simulink model "RADTRANS002"  (R2020b)
settings: Solver=VariableStepAuto  StartTime=0.0  StopTime=10.0  RelTol=1e-3
undefined symbols (not defined in the file): Line_110_C, Line_110_L, Line_110_R, Line_220_C, Line_220_L, Line_220_R, Line_35_C, Line_35_L, Line_35_R, Line_6_L, Line_6_R, Sys_f_Hz, Sys_V_net_kV, Tr_110_35_L_pu, Tr_110_35_R_pu, Tr_110_35_Sn_VA, Tr_110_35_V_HV_kV, Tr_110_35_V_LV_kV, Tr_110_6_L_pu, Tr_110_6_R_pu, Tr_110_6_Sn_VA, Tr_110_6_V_HV_kV, Tr_110_6_V_LV_kV, Tr_220_110_L_pu, Tr_220_110_R_pu, Tr_220_110_Sn_VA, Tr_220_110_V_HV_kV, Tr_220_110_V_LV_kV, Tr_35_04_L_pu, Tr_35_04_R_pu, Tr_35_04_Sn_VA, Tr_35_04_V_HV_kV, Tr_35_04_V_LV_kV, Tr_6_04_L_pu, Tr_6_04_R_pu, Tr_6_04_Sn_VA, Tr_6_04_V_HV_kV, Tr_6_04_V_LV_kV, Ts_powergui
libraries: dspstat3 x288, powerlib x202, powerlib_meascontrol x72
(part 7 of 7)

== system RADTRANS002/M_OUT_Завод_5_1 ==
  Iptg_50 : Display
      settings: Format=bank
  PQptg_50 : Scope  NumInputPorts=2
  "Power0 (3ph, Instantaneous)" : powerlib_meascontrol/Measurements/Power (3ph, Instantaneous)
  Pptg_50 : Display
      settings: Format=bank
  Qptg_50 : Display
      settings: Format=bank
  RMS3 : dspstat3/RMS  run=off  directionMode=Each column  dimension=1  InputProcessing=Columns as channels (frame based)  reset_popup=None
  RMS4 : dspstat3/RMS  run=off  directionMode=Each column  dimension=1  InputProcessing=Columns as channels (frame based)  reset_popup=None
  RMS50 : dspstat3/RMS  run=off  directionMode=Each column  dimension=1  InputProcessing=Columns as channels (frame based)  reset_popup=None
  RMSpt_50 : dspstat3/RMS  run=off  directionMode=Each column  dimension=1  InputProcessing=Columns as channels (frame based)  reset_popup=None
  Real-Ima to Complex : RealImagToComplex
  S : Abs
  SSptg_50 : Scope
  Sptg_50 : Display
      settings: Format=bank
  Three-Phase V-I Measurementpt_50 : powerlib/Measurements/Three-Phase V-I Measurement  VoltageMeasurement=phase-to-ground  SetLabelV=off  LabelV=Vabc  Vpu=off  VpuLL=off  CurrentMeasurement=yes  SetLabelI=off  LabelI=Iabc  Ipu=off  Pbase=100e6  Vbase=500e3  OutputType=Complex  PhasorSimulation=off  PSBequivalent=0
  UIptg_50 : Scope  NumInputPorts=2
  Uptg_50 : Display
      settings: Format=bank
  a : PMIOPort  Side=Right
  b : PMIOPort  Port=2  Side=Right
  c : PMIOPort  Port=3  Side=Right
  A : PMIOPort  Port=4  Side=Left
  B : PMIOPort  Port=5  Side=Left
  C : PMIOPort  Port=6  Side=Left
  tag scope: I_ptg_50=global, P_ptg_50=global, Q_ptg_50=global, S_ptg_50=global, U_ptg_50=global
  wires:
  S/1 -> [S_ptg_50]
  Real-Ima to Complex/1 -> S/1
  [S_ptg_50] -> Sptg_50/1
  [S_ptg_50] -> SSptg_50/1
  [P_ptg_50] -> RMSpt_50/1
  RMSpt_50/1 -> Pptg_50/1
  RMS50/1 -> Qptg_50/1
  [U_ptg_50] -> RMS3/1
  RMS3/1 -> Uptg_50/1
  [P_ptg_50] -> Real-Ima to Complex/1
  [Q_ptg_50] -> RMS50/1
  [I_ptg_50] -> RMS4/1
  RMS4/1 -> Iptg_50/1
  [U_ptg_50] -> UIptg_50/1  "U"
  [P_ptg_50] -> PQptg_50/1  "P"
  [I_ptg_50] -> UIptg_50/2  "I"
  Three-Phase V-I Measurementpt_50/1 -> [U_ptg_50]
  [Q_ptg_50] -> Real-Ima to Complex/2
  Three-Phase V-I Measurementpt_50/2 -> [I_ptg_50]
  [U_ptg_50] -> "Power0 (3ph, Instantaneous)"/1
  [I_ptg_50] -> "Power0 (3ph, Instantaneous)"/2
  "Power0 (3ph, Instantaneous)"/2 -> [Q_ptg_50]
  "Power0 (3ph, Instantaneous)"/1 -> [P_ptg_50]
  [Q_ptg_50] -> PQptg_50/2  "Q"
  connections:
  Three-Phase V-I Measurementpt_50/LConn1 -- A/RConn1
  Three-Phase V-I Measurementpt_50/RConn1 -- a/RConn1
  Three-Phase V-I Measurementpt_50/LConn2 -- B/RConn1
  Three-Phase V-I Measurementpt_50/LConn3 -- C/RConn1
  Three-Phase V-I Measurementpt_50/RConn3 -- c/RConn1
  Three-Phase V-I Measurementpt_50/RConn2 -- b/RConn1

== system RADTRANS002/M_OUT_Завод_5_2 ==
  Iptg_52 : Display
      settings: Format=bank
  PQptg_52 : Scope  NumInputPorts=2
  "Power0 (3ph, Instantaneous)" : powerlib_meascontrol/Measurements/Power (3ph, Instantaneous)
  Pptg_52 : Display
      settings: Format=bank
  Qptg_52 : Display
      settings: Format=bank
  RMS3 : dspstat3/RMS  run=off  directionMode=Each column  dimension=1  InputProcessing=Columns as channels (frame based)  reset_popup=None
  RMS4 : dspstat3/RMS  run=off  directionMode=Each column  dimension=1  InputProcessing=Columns as channels (frame based)  reset_popup=None
  RMS52 : dspstat3/RMS  run=off  directionMode=Each column  dimension=1  InputProcessing=Columns as channels (frame based)  reset_popup=None
  RMSpt_52 : dspstat3/RMS  run=off  directionMode=Each column  dimension=1  InputProcessing=Columns as channels (frame based)  reset_popup=None
  Real-Ima to Complex : RealImagToComplex
  S : Abs
  SSptg_52 : Scope
  Sptg_52 : Display
      settings: Format=bank
  Three-Phase V-I Measurementpt_52 : powerlib/Measurements/Three-Phase V-I Measurement  VoltageMeasurement=phase-to-ground  SetLabelV=off  LabelV=Vabc  Vpu=off  VpuLL=off  CurrentMeasurement=yes  SetLabelI=off  LabelI=Iabc  Ipu=off  Pbase=100e6  Vbase=500e3  OutputType=Complex  PhasorSimulation=off  PSBequivalent=0
  UIptg_52 : Scope  NumInputPorts=2
  Uptg_52 : Display
      settings: Format=bank
  a : PMIOPort  Side=Right
  b : PMIOPort  Port=2  Side=Right
  c : PMIOPort  Port=3  Side=Right
  A : PMIOPort  Port=4  Side=Left
  B : PMIOPort  Port=5  Side=Left
  C : PMIOPort  Port=6  Side=Left
  tag scope: I_ptg_52=global, P_ptg_52=global, Q_ptg_52=global, S_ptg_52=global, U_ptg_52=global
  wires:
  S/1 -> [S_ptg_52]
  Real-Ima to Complex/1 -> S/1
  [S_ptg_52] -> Sptg_52/1
  [S_ptg_52] -> SSptg_52/1
  [P_ptg_52] -> RMSpt_52/1
  RMSpt_52/1 -> Pptg_52/1
  RMS52/1 -> Qptg_52/1
  [U_ptg_52] -> RMS3/1
  RMS3/1 -> Uptg_52/1
  [P_ptg_52] -> Real-Ima to Complex/1
  [Q_ptg_52] -> RMS52/1
  [I_ptg_52] -> RMS4/1
  RMS4/1 -> Iptg_52/1
  [U_ptg_52] -> UIptg_52/1  "U"
  [P_ptg_52] -> PQptg_52/1  "P"
  [I_ptg_52] -> UIptg_52/2  "I"
  Three-Phase V-I Measurementpt_52/1 -> [U_ptg_52]
  [Q_ptg_52] -> Real-Ima to Complex/2
  Three-Phase V-I Measurementpt_52/2 -> [I_ptg_52]
  [U_ptg_52] -> "Power0 (3ph, Instantaneous)"/1
  [I_ptg_52] -> "Power0 (3ph, Instantaneous)"/2
  "Power0 (3ph, Instantaneous)"/2 -> [Q_ptg_52]
  "Power0 (3ph, Instantaneous)"/1 -> [P_ptg_52]
  [Q_ptg_52] -> PQptg_52/2  "Q"
  connections:
  Three-Phase V-I Measurementpt_52/LConn1 -- A/RConn1
  Three-Phase V-I Measurementpt_52/RConn1 -- a/RConn1
  Three-Phase V-I Measurementpt_52/LConn2 -- B/RConn1
  Three-Phase V-I Measurementpt_52/LConn3 -- C/RConn1
  Three-Phase V-I Measurementpt_52/RConn3 -- c/RConn1
  Three-Phase V-I Measurementpt_52/RConn2 -- b/RConn1

== system RADTRANS002/M_OUT_Завод_6_1 ==
  Iptg_62 : Display
      settings: Format=bank
  PQptg_62 : Scope  NumInputPorts=2
  "Power0 (3ph, Instantaneous)" : powerlib_meascontrol/Measurements/Power (3ph, Instantaneous)
  Pptg_62 : Display
      settings: Format=bank
  Qptg_62 : Display
      settings: Format=bank
  RMS3 : dspstat3/RMS  run=off  directionMode=Each column  dimension=1  InputProcessing=Columns as channels (frame based)  reset_popup=None
  RMS4 : dspstat3/RMS  run=off  directionMode=Each column  dimension=1  InputProcessing=Columns as channels (frame based)  reset_popup=None
  RMS62 : dspstat3/RMS  run=off  directionMode=Each column  dimension=1  InputProcessing=Columns as channels (frame based)  reset_popup=None
  RMSpt_62 : dspstat3/RMS  run=off  directionMode=Each column  dimension=1  InputProcessing=Columns as channels (frame based)  reset_popup=None
  Real-Ima to Complex : RealImagToComplex
  S : Abs
  SSptg_62 : Scope
  Sptg_62 : Display
      settings: Format=bank
  Three-Phase V-I Measurementpt_62 : powerlib/Measurements/Three-Phase V-I Measurement  VoltageMeasurement=phase-to-ground  SetLabelV=off  LabelV=Vabc  Vpu=off  VpuLL=off  CurrentMeasurement=yes  SetLabelI=off  LabelI=Iabc  Ipu=off  Pbase=100e6  Vbase=500e3  OutputType=Complex  PhasorSimulation=off  PSBequivalent=0
  UIptg_62 : Scope  NumInputPorts=2
  Uptg_62 : Display
      settings: Format=bank
  a : PMIOPort  Side=Right
  b : PMIOPort  Port=2  Side=Right
  c : PMIOPort  Port=3  Side=Right
  A : PMIOPort  Port=4  Side=Left
  B : PMIOPort  Port=5  Side=Left
  C : PMIOPort  Port=6  Side=Left
  tag scope: I_ptg_62=global, P_ptg_62=global, Q_ptg_62=global, S_ptg_62=global, U_ptg_62=global
  wires:
  S/1 -> [S_ptg_62]
  Real-Ima to Complex/1 -> S/1
  [S_ptg_62] -> Sptg_62/1
  [S_ptg_62] -> SSptg_62/1
  [P_ptg_62] -> RMSpt_62/1
  RMSpt_62/1 -> Pptg_62/1
  RMS62/1 -> Qptg_62/1
  [U_ptg_62] -> RMS3/1
  RMS3/1 -> Uptg_62/1
  [P_ptg_62] -> Real-Ima to Complex/1
  [Q_ptg_62] -> RMS62/1
  [I_ptg_62] -> RMS4/1
  RMS4/1 -> Iptg_62/1
  [U_ptg_62] -> UIptg_62/1  "U"
  [P_ptg_62] -> PQptg_62/1  "P"
  [I_ptg_62] -> UIptg_62/2  "I"
  Three-Phase V-I Measurementpt_62/1 -> [U_ptg_62]
  [Q_ptg_62] -> Real-Ima to Complex/2
  Three-Phase V-I Measurementpt_62/2 -> [I_ptg_62]
  [U_ptg_62] -> "Power0 (3ph, Instantaneous)"/1
  [I_ptg_62] -> "Power0 (3ph, Instantaneous)"/2
  "Power0 (3ph, Instantaneous)"/2 -> [Q_ptg_62]
  "Power0 (3ph, Instantaneous)"/1 -> [P_ptg_62]
  [Q_ptg_62] -> PQptg_62/2  "Q"
  connections:
  Three-Phase V-I Measurementpt_62/LConn1 -- A/RConn1
  Three-Phase V-I Measurementpt_62/RConn1 -- a/RConn1
  Three-Phase V-I Measurementpt_62/LConn2 -- B/RConn1
  Three-Phase V-I Measurementpt_62/LConn3 -- C/RConn1
  Three-Phase V-I Measurementpt_62/RConn3 -- c/RConn1
  Three-Phase V-I Measurementpt_62/RConn2 -- b/RConn1

== system RADTRANS002/M_OUT_Завод_6_2 ==
  Iptg_64 : Display
      settings: Format=bank
  PQptg_64 : Scope  NumInputPorts=2
  "Power0 (3ph, Instantaneous)" : powerlib_meascontrol/Measurements/Power (3ph, Instantaneous)
  Pptg_64 : Display
      settings: Format=bank
  Qptg_64 : Display
      settings: Format=bank
  RMS3 : dspstat3/RMS  run=off  directionMode=Each column  dimension=1  InputProcessing=Columns as channels (frame based)  reset_popup=None
  RMS4 : dspstat3/RMS  run=off  directionMode=Each column  dimension=1  InputProcessing=Columns as channels (frame based)  reset_popup=None
  RMS64 : dspstat3/RMS  run=off  directionMode=Each column  dimension=1  InputProcessing=Columns as channels (frame based)  reset_popup=None
  RMSpt_64 : dspstat3/RMS  run=off  directionMode=Each column  dimension=1  InputProcessing=Columns as channels (frame based)  reset_popup=None
  Real-Ima to Complex : RealImagToComplex
  S : Abs
  SSptg_64 : Scope
  Sptg_64 : Display
      settings: Format=bank
  Three-Phase V-I Measurementpt_64 : powerlib/Measurements/Three-Phase V-I Measurement  VoltageMeasurement=phase-to-ground  SetLabelV=off  LabelV=Vabc  Vpu=off  VpuLL=off  CurrentMeasurement=yes  SetLabelI=off  LabelI=Iabc  Ipu=off  Pbase=100e6  Vbase=500e3  OutputType=Complex  PhasorSimulation=off  PSBequivalent=0
  UIptg_64 : Scope  NumInputPorts=2
  Uptg_64 : Display
      settings: Format=bank
  a : PMIOPort  Side=Right
  b : PMIOPort  Port=2  Side=Right
  c : PMIOPort  Port=3  Side=Right
  A : PMIOPort  Port=4  Side=Left
  B : PMIOPort  Port=5  Side=Left
  C : PMIOPort  Port=6  Side=Left
  tag scope: I_ptg_64=global, P_ptg_64=global, Q_ptg_64=global, S_ptg_64=global, U_ptg_64=global
  wires:
  S/1 -> [S_ptg_64]
  Real-Ima to Complex/1 -> S/1
  [S_ptg_64] -> Sptg_64/1
  [S_ptg_64] -> SSptg_64/1
  [P_ptg_64] -> RMSpt_64/1
  RMSpt_64/1 -> Pptg_64/1
  RMS64/1 -> Qptg_64/1
  [U_ptg_64] -> RMS3/1
  RMS3/1 -> Uptg_64/1
  [P_ptg_64] -> Real-Ima to Complex/1
  [Q_ptg_64] -> RMS64/1
  [I_ptg_64] -> RMS4/1
  RMS4/1 -> Iptg_64/1
  [U_ptg_64] -> UIptg_64/1  "U"
  [P_ptg_64] -> PQptg_64/1  "P"
  [I_ptg_64] -> UIptg_64/2  "I"
  Three-Phase V-I Measurementpt_64/1 -> [U_ptg_64]
  [Q_ptg_64] -> Real-Ima to Complex/2
  Three-Phase V-I Measurementpt_64/2 -> [I_ptg_64]
  [U_ptg_64] -> "Power0 (3ph, Instantaneous)"/1
  [I_ptg_64] -> "Power0 (3ph, Instantaneous)"/2
  "Power0 (3ph, Instantaneous)"/2 -> [Q_ptg_64]
  "Power0 (3ph, Instantaneous)"/1 -> [P_ptg_64]
  [Q_ptg_64] -> PQptg_64/2  "Q"
  connections:
  Three-Phase V-I Measurementpt_64/LConn1 -- A/RConn1
  Three-Phase V-I Measurementpt_64/RConn1 -- a/RConn1
  Three-Phase V-I Measurementpt_64/LConn2 -- B/RConn1
  Three-Phase V-I Measurementpt_64/LConn3 -- C/RConn1
  Three-Phase V-I Measurementpt_64/RConn3 -- c/RConn1
  Three-Phase V-I Measurementpt_64/RConn2 -- b/RConn1
